simulink model "untitled"  (Simulink 7.5)
settings: Solver=ode45  StartTime=0.0  StopTime=inf  MaxStep=0.01  RelTol=1e-3
settings Model: Creator=psoltysiak  LastModifiedBy=Soltys
settings DebuggingCC: StrictBusMsg=Warning

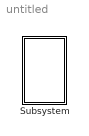
== system untitled ==
  Subsystem : Subsystem  mask{l1=3, l2=2, m1=10, m2=5, k1=1, k2=1, phi1=45, phi2=60, g=9.81, to=0.1}
      mask prompts: l1 "dlugosc wahadla 1"; l2 "dlugosc wahadla 2"; m1 "masa 1"; m2 "masa 2"; k1 "wsp. tlumienia 1"; k2 "wsp. tlumienia 2"; phi1 "wychwychylenie 1"; phi2 "wychylenie 2"; g "przys. ziemskie"; to "czas. odswiezania"

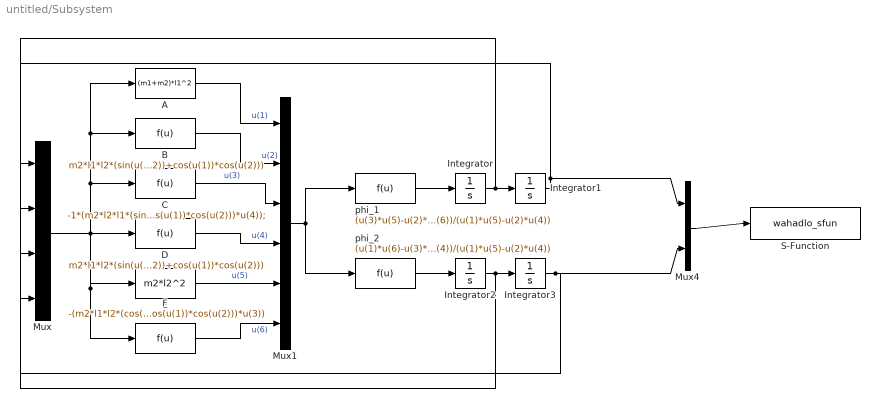
== system untitled/Subsystem ==
  A : Fcn  Expr=(m1+m2)*l1^2
  B : Fcn  Expr=m2*l1*l2*(sin(u(1))*sin(u(2))+cos(u(1))*cos(u(2)))
  C : Fcn  Expr=-1*(m2*l2*l1*(sin(u(1))*cos(u(2))-cos(u(1))*sin(u(2)))*u(4)+(m1+m2)*g*l1*sin(u(1))+k1*l1^2*u(3)+k2*l1*l2*(sin(u(1))*sin(u(2))+cos(u(1))*cos(u(2)))*u(4));
  D : Fcn  Expr=m2*l1*l2*(sin(u(1))*sin(u(2))+cos(u(1))*cos(u(2)))
  E : Fcn  Expr=m2*l2^2
  F : Fcn  Expr=-(m2*l1*l2*(cos(u(1))*sin(u(2))-sin(u(1))*cos(u(2)))*u(3)^2+m2*g*l2*sin(u(2))+k2*l2^2*u(4)+k2*l1*l2*(sin(u(1))*sin(u(2))+cos(u(1))*cos(u(2)))*u(3))
  Integrator : Integrator
  Integrator1 : Integrator  InitialCondition=phi1*pi/180
  Integrator2 : Integrator
  Integrator3 : Integrator  InitialCondition=phi2*pi/180
  Mux : Mux
  Mux1 : Mux  Inputs=6
  Mux4 : Mux  Inputs=2
  S-Function : S-Function  FunctionName=wahadlo_sfun  Parameters=l1,l2,m1,m2,phi1,phi2,to  EnableBusSupport=off
  phi_1 : Fcn  Expr=(u(3)*u(5)-u(2)*u(6))/(u(1)*u(5)-u(2)*u(4))
  phi_2 : Fcn  Expr=(u(1)*u(6)-u(3)*u(4))/(u(1)*u(5)-u(2)*u(4))
  wires:
  Mux/1 -> D/1, C/1, B/1, A/1, F/1, E/1
  A/1 -> Mux1/1  "u(1)"
  B/1 -> Mux1/2  "u(2)"
  C/1 -> Mux1/3  "u(3)"
  D/1 -> Mux1/4  "u(4)"
  E/1 -> Mux1/5  "u(5)"
  F/1 -> Mux1/6  "u(6)"
  Mux1/1 -> phi_1/1, phi_2/1
  phi_1/1 -> Integrator/1
  Integrator/1 -> Integrator1/1, Mux/3
  phi_2/1 -> Integrator2/1
  Integrator2/1 -> Integrator3/1, Mux/4
  Integrator1/1 -> Mux/1, Mux4/1
  Integrator3/1 -> Mux/2, Mux4/2
  Mux4/1 -> S-Function/1
